simulink model "lab7_inciso2"  (R2021a)
settings: Solver=VariableStepAuto  StartTime=0.0  StopTime=F  RelTol=1e-3
values from neighbouring files (symbols this model uses):
  A3 = [(-1*(r1+r2)/(r1*r2*c1)), (1/(r2*c1)), -1/(r2*c1); 0,0, -1/(r3*c2); -1/(r2*c3),1/(r2*c3), -1*(r2+r3)/(r2*r3*c3)]    [Lab7.m]
  Acl_tercero = A3-B3*Kpp    [Lab7.m]
  B3 = [1/(r1*c1);0;0]    [Lab7.m]
  C3 = [0,1,0]    [Lab7.m]
  Kpp = place(A3,B3,p)    [Lab7.m]
  Lpp = place(A3',C3',p_L)'    [Lab7.m]
  Nbar_tercero = rscale(sys,Kpp)    [Lab7.m]
  T = 1/0.667    (= 1.49925037481)    [Lab7.m]
settings Model: Creator=fersa  LastModifiedBy=fersa

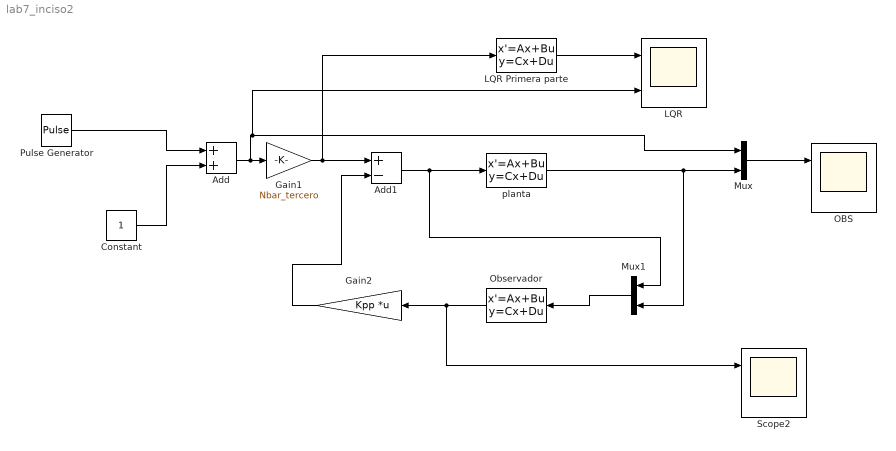
== system lab7_inciso2 ==
  Add : Sum
  Add1 : Sum  Inputs=+-
  Constant : Constant
  Gain1 : Gain  Gain=Nbar_tercero
  Gain2 : Gain  Gain=Kpp  Multiplication=Matrix(K*u) (u vector)
  LQR : Scope  NumInputPorts=2
  LQR Primera parte : StateSpace  A=Acl_tercero  B=B3  C=C3  D=0  InitialCondition=0  ParameterTunability=Unconstrained
  Mux : Mux  Inputs=2
  Mux1 : Mux  Inputs=2
  OBS : Scope  NumInputPorts=2
  Observador : StateSpace  A=A3-Lpp*C3  B=[B3 Lpp]  C=[1 0 0; 0 1 0; 0 0 1]  D=zeros(3,2)  InitialCondition=0  ParameterTunability=Unconstrained
  Pulse Generator : DiscretePulseGenerator  PulseType=Time based  Period=T  PulseWidth=50  PhaseDelay=0.75
  Scope2 : Scope  NumInputPorts=2
  planta : StateSpace  A=A3  B=B3  C=C3  D=0  InitialCondition=0  ParameterTunability=Unconstrained
  wires:
  LQR Primera parte/1 -> LQR/1
  Pulse Generator/1 -> Add/1
  Constant/1 -> Add/2
  Add/1 -> LQR/2, Mux/1, Gain1/1
  Gain1/1 -> LQR Primera parte/1, Add1/1
  Add1/1 -> Mux1/1, planta/1
  planta/1 -> Mux1/2, Mux/2
  Mux/1 -> OBS/1
  Observador/1 -> Scope2/1, Gain2/1
  Gain2/1 -> Add1/2
  Mux1/1 -> Observador/1
